simulink model "simLAB"  (R2017a)
settings: Solver=VariableStepAuto  StartTime=0.0  StopTime=60  RelTol=1e-3
libraries: cstblocks x6
settings Model: Creator=Administrator  LastModifiedBy=xinjiay

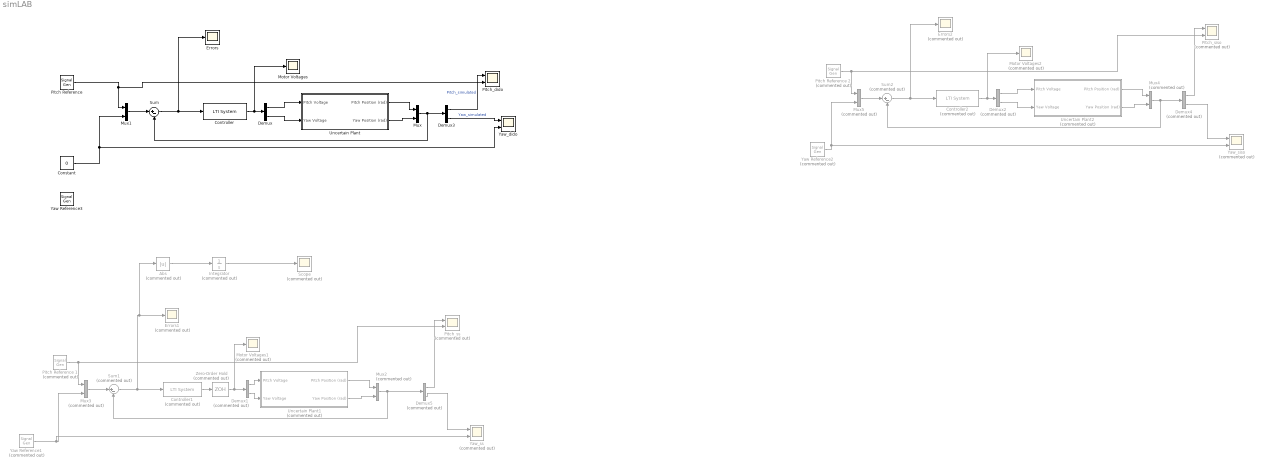
== system simLAB ==
  Abs : Abs  Commented=on
  Constant : Constant  Value=0
  Controller : cstblocks/LTI System  sys=K_loop_siso  IC=[]
  Controller1 : cstblocks/LTI System  Commented=on  sys=K_loop_dido_ss  IC=[]
  Controller2 : cstblocks/LTI System  Commented=on  sys=K_loop_siso  IC=[]
  Demux : Demux  Outputs=2
  Demux{1..2,4..5} (4 alike) : Demux  Commented=on  Outputs=2
  Demux3 : Demux  Outputs=2
  Errors : Scope
  Errors1 : Scope  Commented=on
  Errors2 : Scope  Commented=on
  Integrator : Integrator  Commented=on
  Motor Voltages : Scope
  Motor Voltages1 : Scope  Commented=on
  Motor Voltages2 : Scope  Commented=on
  Mux : Mux  Inputs=2
  Mux1 : Mux  Inputs=2
  Mux{2..5} (4 alike) : Mux  Commented=on  Inputs=2
  Pitch Reference : SignalGenerator  WaveForm=square  Amplitude=pi/6  Frequency=0.4  Units=rad/sec
  Pitch Reference 1 : SignalGenerator  Commented=on  WaveForm=square  Amplitude=pi/6  Frequency=0.4  Units=rad/sec
  Pitch Reference 2 : SignalGenerator  Commented=on  WaveForm=square  Amplitude=pi/6  Frequency=0.4  Units=rad/sec
  Pitch_dido : Scope  NumInputPorts=2
  Pitch_siso : Scope  Commented=on  NumInputPorts=2
  Pitch_ss : Scope  Commented=on  NumInputPorts=2
  Scope : Scope  Commented=on
  Sum : Sum  Inputs=|+-
  Sum1 : Sum  Commented=on  Inputs=|+-
  Sum2 : Sum  Commented=on  Inputs=|+-
  Uncertain Plant : Subsystem
  Uncertain Plant1 : Subsystem  Commented=on
  Uncertain Plant2 : Subsystem  Commented=on
  Yaw Reference1 : SignalGenerator  Commented=on  WaveForm=square  Amplitude=pi/4  Frequency=0.5  Units=rad/sec
  Yaw Reference2 : SignalGenerator  Commented=on  WaveForm=square  Amplitude=pi/4  Frequency=0.5  Units=rad/sec
  Yaw Reference3 : SignalGenerator  WaveForm=square  Amplitude=pi/4  Frequency=0.5  Units=rad/sec
  Yaw_dido : Scope  NumInputPorts=2
  Yaw_siso : Scope  Commented=on  NumInputPorts=2
  Yaw_ss : Scope  Commented=on  NumInputPorts=2
  Zero-Order Hold : ZeroOrderHold  Commented=on  SampleTime=0.002
  wires:
  Mux1/1 -> Sum/1
  Pitch Reference/1 -> Pitch_dido/2, Mux1/1
  Uncertain Plant/1(Pitch Position (rad)) -> Mux/1
  Sum/1 -> Errors/1, Controller/1
  Demux/1 -> Uncertain Plant/1(Pitch Voltage)
  Uncertain Plant/2(Yaw Position (rad)) -> Mux/2
  Demux/2 -> Uncertain Plant/2(Yaw Voltage)
  Controller/1 -> Motor Voltages/1, Demux/1
  Mux/1 -> Demux3/1, Sum/2
  Constant/1 -> Mux1/2, Yaw_dido/2
  Uncertain Plant1/1(Pitch Position (rad)) -> Mux2/1
  Sum1/1 -> Abs/1, Errors1/1, Controller1/1
  Uncertain Plant1/2(Yaw Position (rad)) -> Mux2/2
  Demux1/2 -> Uncertain Plant1/2(Yaw Voltage)
  Mux3/1 -> Sum1/1
  Demux1/1 -> Uncertain Plant1/1(Pitch Voltage)
  Controller1/1 -> Zero-Order Hold/1
  Zero-Order Hold/1 -> Motor Voltages1/1, Demux1/1
  Yaw Reference2/1 -> Yaw_siso/2, Mux5/2
  Uncertain Plant2/1(Pitch Position (rad)) -> Mux4/1
  Controller2/1 -> Motor Voltages2/1, Demux2/1
  Sum2/1 -> Errors2/1, Controller2/1
  Demux2/2 -> Uncertain Plant2/2(Yaw Voltage)
  Mux4/1 -> Demux4/1, Sum2/2
  Mux5/1 -> Sum2/1
  Demux2/1 -> Uncertain Plant2/1(Pitch Voltage)
  Pitch Reference 2/1 -> Pitch_siso/2, Mux5/1
  Uncertain Plant2/2(Yaw Position (rad)) -> Mux4/2
  Demux3/1 -> Pitch_dido/1  "Pitch_simulated"
  Demux3/2 -> Yaw_dido/1  "Yaw_simulated"
  Demux4/1 -> Pitch_siso/1
  Demux4/2 -> Yaw_siso/1
  Yaw Reference1/1 -> Yaw_ss/2, Mux3/2
  Mux2/1 -> Demux5/1, Sum1/2
  Demux5/2 -> Yaw_ss/1
  Demux5/1 -> Pitch_ss/1
  Pitch Reference 1/1 -> Pitch_ss/2, Mux3/1
  Integrator/1 -> Scope/1
  Abs/1 -> Integrator/1

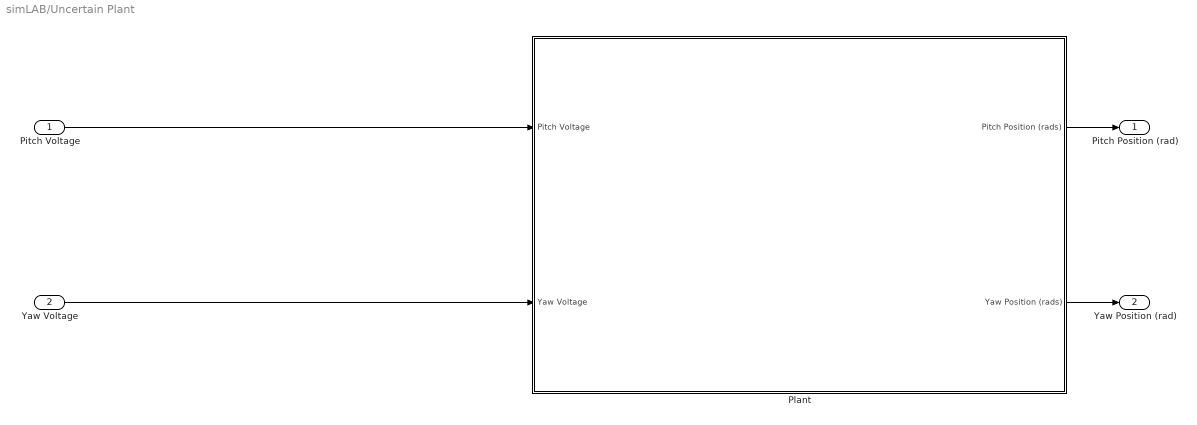
== system simLAB/Uncertain Plant ==
  Pitch Voltage : Inport
  Yaw Voltage : Inport  Port=2
  Plant : Subsystem
  Pitch Position (rad) : Outport
  Yaw Position (rad) : Outport  Port=2
  wires:
  Pitch Voltage/1 -> Plant/1(Pitch Voltage)
  Yaw Voltage/1 -> Plant/2(Yaw Voltage)
  Plant/1(Pitch Position (rads)) -> Pitch Position (rad)/1
  Plant/2(Yaw Position (rads)) -> Yaw Position (rad)/1

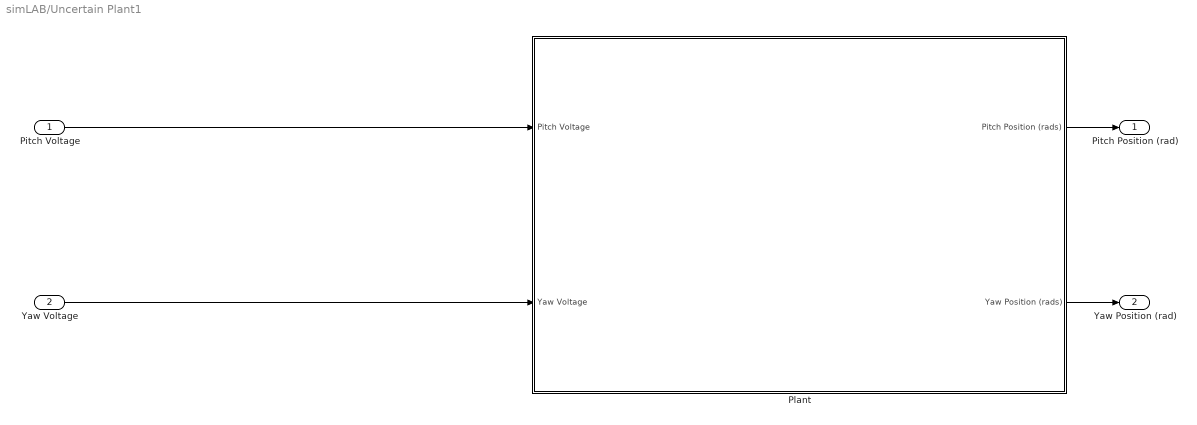
== system simLAB/Uncertain Plant1 ==
  Pitch Voltage : Inport
  Yaw Voltage : Inport  Port=2
  Plant : Subsystem
  Pitch Position (rad) : Outport
  Yaw Position (rad) : Outport  Port=2
  wires:
  Pitch Voltage/1 -> Plant/1(Pitch Voltage)
  Yaw Voltage/1 -> Plant/2(Yaw Voltage)
  Plant/1(Pitch Position (rads)) -> Pitch Position (rad)/1
  Plant/2(Yaw Position (rads)) -> Yaw Position (rad)/1

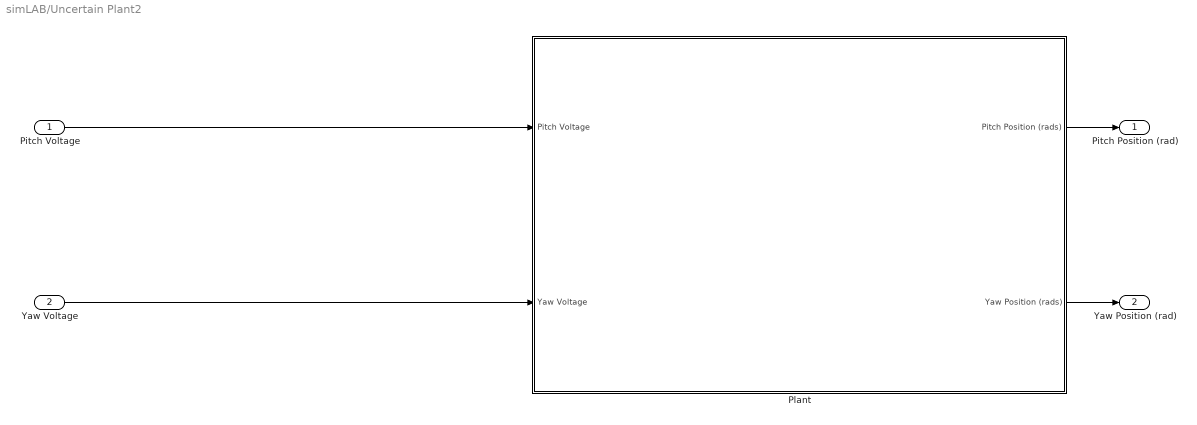
== system simLAB/Uncertain Plant2 ==
  Pitch Voltage : Inport
  Yaw Voltage : Inport  Port=2
  Plant : Subsystem
  Pitch Position (rad) : Outport
  Yaw Position (rad) : Outport  Port=2
  wires:
  Pitch Voltage/1 -> Plant/1(Pitch Voltage)
  Yaw Voltage/1 -> Plant/2(Yaw Voltage)
  Plant/1(Pitch Position (rads)) -> Pitch Position (rad)/1
  Plant/2(Yaw Position (rads)) -> Yaw Position (rad)/1

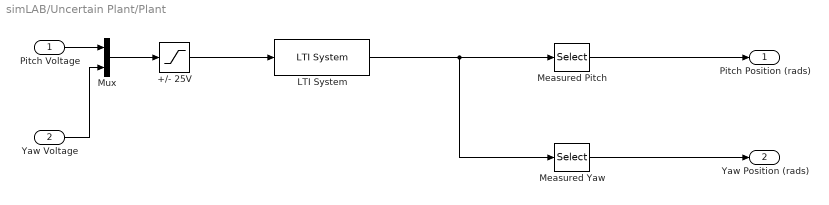
== system simLAB/Uncertain Plant/Plant ==
  Pitch Voltage : Inport
  Yaw Voltage : Inport  Port=2
  +/- 25V : Saturate  UpperLimit=25  LowerLimit=-25
  LTI System : cstblocks/LTI System  sys=G  IC=[]
  Measured Pitch : Selector  InputPortWidth=2  IndexOptions=Index vector (dialog)  Indices=[1]  OutputSizes=1
  Measured Yaw : Selector  InputPortWidth=2  IndexOptions=Index vector (dialog)  Indices=[2]  OutputSizes=1
  Mux : Mux  Inputs=2
  Pitch Position (rads) : Outport
  Yaw Position (rads) : Outport  Port=2
  wires:
  Pitch Voltage/1 -> Mux/1
  Yaw Voltage/1 -> Mux/2
  Mux/1 -> +/- 25V/1
  Measured Yaw/1 -> Yaw Position (rads)/1
  +/- 25V/1 -> LTI System/1
  LTI System/1 -> Measured Pitch/1, Measured Yaw/1
  Measured Pitch/1 -> Pitch Position (rads)/1

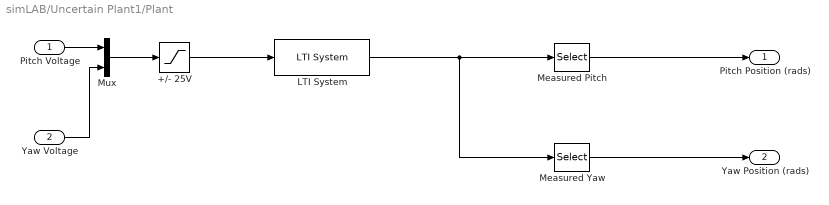
== system simLAB/Uncertain Plant1/Plant ==
  Pitch Voltage : Inport
  Yaw Voltage : Inport  Port=2
  +/- 25V : Saturate  UpperLimit=25  LowerLimit=-25
  LTI System : cstblocks/LTI System  sys=G  IC=[]
  Measured Pitch : Selector  InputPortWidth=2  IndexOptions=Index vector (dialog)  Indices=[1]  OutputSizes=1
  Measured Yaw : Selector  InputPortWidth=2  IndexOptions=Index vector (dialog)  Indices=[2]  OutputSizes=1
  Mux : Mux  Inputs=2
  Pitch Position (rads) : Outport
  Yaw Position (rads) : Outport  Port=2
  wires:
  Pitch Voltage/1 -> Mux/1
  Yaw Voltage/1 -> Mux/2
  Mux/1 -> +/- 25V/1
  Measured Yaw/1 -> Yaw Position (rads)/1
  +/- 25V/1 -> LTI System/1
  LTI System/1 -> Measured Pitch/1, Measured Yaw/1
  Measured Pitch/1 -> Pitch Position (rads)/1

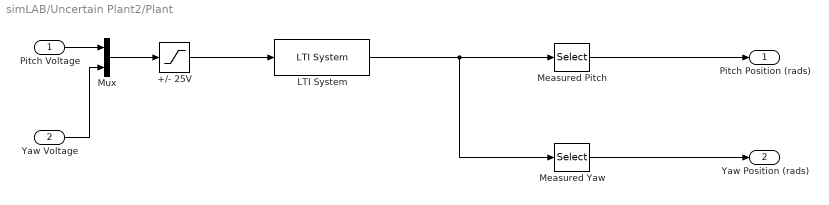
== system simLAB/Uncertain Plant2/Plant ==
  Pitch Voltage : Inport
  Yaw Voltage : Inport  Port=2
  +/- 25V : Saturate  UpperLimit=25  LowerLimit=-25
  LTI System : cstblocks/LTI System  sys=G  IC=[]
  Measured Pitch : Selector  InputPortWidth=2  IndexOptions=Index vector (dialog)  Indices=[1]  OutputSizes=1
  Measured Yaw : Selector  InputPortWidth=2  IndexOptions=Index vector (dialog)  Indices=[2]  OutputSizes=1
  Mux : Mux  Inputs=2
  Pitch Position (rads) : Outport
  Yaw Position (rads) : Outport  Port=2
  wires:
  Pitch Voltage/1 -> Mux/1
  Yaw Voltage/1 -> Mux/2
  Mux/1 -> +/- 25V/1
  Measured Yaw/1 -> Yaw Position (rads)/1
  +/- 25V/1 -> LTI System/1
  LTI System/1 -> Measured Pitch/1, Measured Yaw/1
  Measured Pitch/1 -> Pitch Position (rads)/1
